simulink model "lht_1280_720"  (R2020a)
settings: Solver=FixedStepDiscrete  StartTime=0.0  StopTime=inf  RelTol=1e-3
InitFcn:
  | setup_parallel_hough_transform;
StopFcn:
  | stop_parallel_hough_accumulator;
values from neighbouring files (symbols this model uses):
  bitsRho = ceil(log2(maxRho*2))    [setup_parallel_hough_transform.m]
  height = 720    [setup_parallel_hough_transform.m]
  inarray = uint8(fi(edge, 0, 1, 0))    [setup_parallel_hough_transform.m]
  width = 1280    [setup_parallel_hough_transform.m]
undefined symbols (not defined in the file or in its folder): fclk, nTheta
libraries: hdlsllib x15, simulink x12, dspsrcs4 x1
(part 1 of 2)
settings Model: DataTypeOverride=Off  SimulationMode=rapid-accelerator  Creator=david  LastModifiedBy=david
settings OptimizationCC: BlockReduction=off  ConditionallyExecuteInputs=off  DefaultParameterBehavior=Inlined
settings DebuggingCC: AlgebraicLoopMsg=error  SingleTaskRateTransMsg=error
settings HardwareCC: ProdBitPerPointer=32  ProdBitPerSizeT=32  ProdBitPerPtrDiffT=32  ProdLargestAtomicFloat=None  ProdIntDivRoundTo=Undefined  ProdEndianess=Unspecified  ProdWordSize=32  ProdHWDeviceType=ASIC/FPGA->ASIC/FPGA  TargetBitPerPointer=64  TargetBitPerSizeT=64  TargetBitPerPtrDiffT=64  TargetLongLongMode=on  TargetIntDivRoundTo=Zero  TargetEndianess=LittleEndian  TargetWordSize=64  TargetHWDeviceType=Custom Processor->MATLAB Host Computer  ProdEqTarget=off

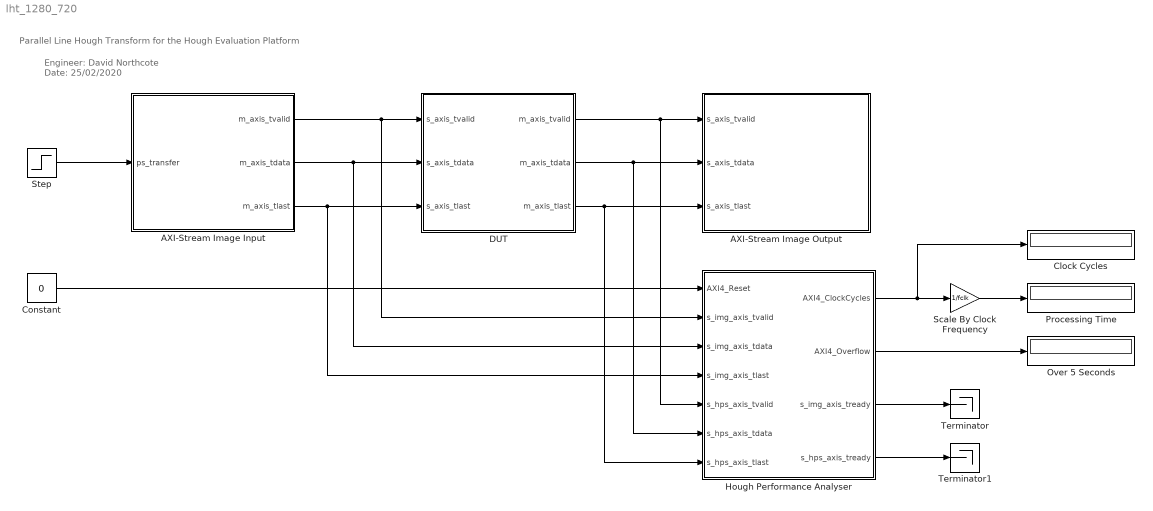
== system lht_1280_720 ==
  note: Engineer: David Northcote
      | Date: 25/02/2020
  note: Parallel Line Hough Transform for the Hough Evaluation Platform
  AXI-Stream Image Input : Subsystem  mask{image=inarray, clk=1/fclk}
      mask prompts: image "Input Image:"; clk "Clock Rate:"
      mask init:
      | [height, width] = size(image);
      mask DialogControl DescGroupVar Prompt: AXI-Stream Image Input
      mask DialogControl DescTextVar Prompt: This block simulates an AXI-Stream image input for interfacing to a hardware accelerator or IP Core.
      mask DialogControl ParameterGroupVar Prompt: Main
  AXI-Stream Image Output : Subsystem  mask{height=ceil(sqrt((height/2)^2+(width/2)^2))*2, width=numel([0:1:179]), clk=1/fclk, d=0}
      mask prompts: height "Image Height:"; width "Image Width:"; clk "Clock Rate:"; d "Frame Capture Number"
      mask DialogControl DescGroupVar Prompt: AXI-Stream Image Output
      mask DialogControl DescTextVar Prompt: Image output using the AXI-Stream interface. Simulates an AXI DMA write channel.
      mask DialogControl ParameterGroupVar Prompt: Main
  Clock Cycles : Display
  Constant : Constant  Value=0  OutDataTypeStr=boolean  SampleTime=1/fclk
  DUT : Subsystem  TreatAsAtomicUnit=on
  Hough Performance Analyser : Subsystem  TreatAsAtomicUnit=on
  Over 5 Seconds : Display
  Processing Time : Display
  Scale By Clock Frequency : Gain  Gain=1/fclk  ParamDataTypeStr=double  OutDataTypeStr=double
  Step : Step  Time=2/150e6  SampleTime=1/fclk
  Terminator : Terminator
  Terminator1 : Terminator
  wires:
  Hough Performance Analyser/1(AXI4_ClockCycles) -> Clock Cycles/1, Scale By Clock Frequency/1
  Scale By Clock Frequency/1 -> Processing Time/1
  DUT/3(m_axis_tlast) -> Hough Performance Analyser/7(s_hps_axis_tlast), AXI-Stream Image Output/3(s_axis_tlast)
  DUT/2(m_axis_tdata) -> Hough Performance Analyser/6(s_hps_axis_tdata), AXI-Stream Image Output/2(s_axis_tdata)
  DUT/1(m_axis_tvalid) -> Hough Performance Analyser/5(s_hps_axis_tvalid), AXI-Stream Image Output/1(s_axis_tvalid)
  AXI-Stream Image Input/3(m_axis_tlast) -> DUT/3(s_axis_tlast), Hough Performance Analyser/4(s_img_axis_tlast)
  AXI-Stream Image Input/1(m_axis_tvalid) -> DUT/1(s_axis_tvalid), Hough Performance Analyser/2(s_img_axis_tvalid)
  AXI-Stream Image Input/2(m_axis_tdata) -> DUT/2(s_axis_tdata), Hough Performance Analyser/3(s_img_axis_tdata)
  Hough Performance Analyser/2(AXI4_Overflow) -> Over 5 Seconds/1
  Constant/1 -> Hough Performance Analyser/1(AXI4_Reset)
  Step/1 -> AXI-Stream Image Input/1(ps_transfer)
  Hough Performance Analyser/4(s_hps_axis_tready) -> Terminator1/1
  Hough Performance Analyser/3(s_img_axis_tready) -> Terminator/1

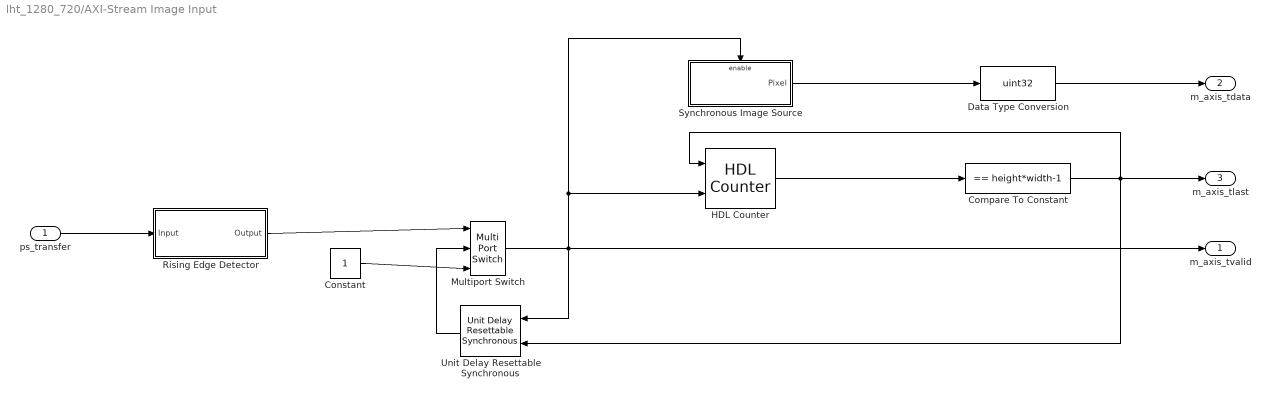
== system lht_1280_720/AXI-Stream Image Input ==
  ps_transfer : Inport
  Compare To Constant : simulink/Logic and Bit Operations/Compare To Constant  relop===  const=height*width-1  OutDataTypeStr=boolean
  Constant : Constant  OutDataTypeStr=boolean  SampleTime=-1
  Data Type Conversion : DataTypeConversion  OutDataTypeStr=uint32
  HDL Counter : hdlsllib/Sources/HDL Counter  CountType=Free running  CountInit=0  CountStep=1  CountMax=width*height-1  CountFromType=Initial value  CountFrom=0  CountResetPort=on  CountLoadPort=off  CountEnbPort=on  CountDirPort=off  CountDataType=Unsigned  CountWordLen=32  CountFracLen=0  CountSampTime=1
  Multiport Switch : MultiPortSwitch  DataPortOrder=Zero-based contiguous  Inputs=2  zeroidx=on
  Rising Edge Detector : Subsystem
  Synchronous Image Source : Subsystem
  Unit Delay Resettable Synchronous : hdlsllib/Discrete/Unit Delay Resettable Synchronous  InitialCondition=0.0  SampleTime=-1
      settings: SourceProductBaseCode=SL
  m_axis_tvalid : Outport
  m_axis_tdata : Outport  Port=2
  m_axis_tlast : Outport  Port=3
  wires:
  Constant/1 -> Multiport Switch/3
  Rising Edge Detector/1(Output) -> Multiport Switch/1
  Unit Delay Resettable Synchronous/1 -> Multiport Switch/2
  ps_transfer/1 -> Rising Edge Detector/1(Input)
  Data Type Conversion/1 -> m_axis_tdata/1
  Compare To Constant/1 -> m_axis_tlast/1, HDL Counter/1, Unit Delay Resettable Synchronous/2
  Multiport Switch/1 -> m_axis_tvalid/1, Synchronous Image Source/Enable, HDL Counter/2, Unit Delay Resettable Synchronous/1
  Synchronous Image Source/1(Pixel) -> Data Type Conversion/1
  HDL Counter/1 -> Compare To Constant/1

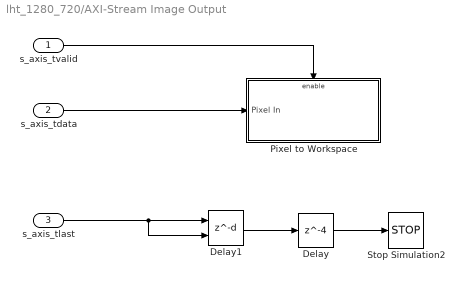
== system lht_1280_720/AXI-Stream Image Output ==
  s_axis_tvalid : Inport
  s_axis_tdata : Inport  Port=2
  s_axis_tlast : Inport  Port=3
  Delay : Delay  DelayLength=4
  Delay1 : Delay  DelayLength=d  ShowEnablePort=on
      settings: InputPortMap=u0,e6
  Pixel to Workspace : Subsystem
  Stop Simulation2 : Stop
  wires:
  Delay/1 -> Stop Simulation2/1
  Delay1/1 -> Delay/1
  s_axis_tlast/1 -> Delay1/1, Delay1/2
  s_axis_tdata/1 -> Pixel to Workspace/1(Pixel In)
  s_axis_tvalid/1 -> Pixel to Workspace/Enable

== system lht_1280_720/DUT ==
  s_axis_tvalid : Inport
  s_axis_tdata : Inport  Port=2
  s_axis_tlast : Inport  Port=3
  LHT : Subsystem
  m_axis_tvalid : Outport  VectorParamsAs1DForOutWhenUnconnected=off
  m_axis_tdata : Outport  Port=2  VectorParamsAs1DForOutWhenUnconnected=off
  m_axis_tlast : Outport  Port=3  VectorParamsAs1DForOutWhenUnconnected=off
  wires:
  s_axis_tdata/1 -> LHT/1(s_tdata)
  s_axis_tvalid/1 -> LHT/2(s_tvalid)
  s_axis_tlast/1 -> LHT/3(s_tlast)
  LHT/3(m_axis_tlast) -> m_axis_tlast/1
  LHT/1(m_axis_tdata) -> m_axis_tdata/1
  LHT/2(m_axis_tvalid) -> m_axis_tvalid/1

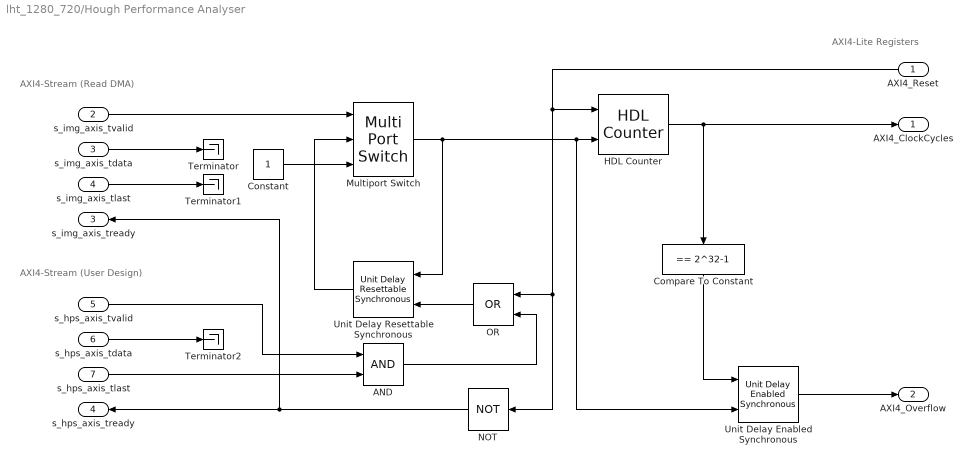
== system lht_1280_720/Hough Performance Analyser ==
  note: AXI4-Stream (Read DMA)
  note: AXI4-Stream (User Design)
  note: AXI4-Lite Registers
  AXI4_Reset : Inport
  s_img_axis_tvalid : Inport  Port=2
  s_img_axis_tdata : Inport  Port=3
  s_img_axis_tlast : Inport  Port=4
  s_hps_axis_tvalid : Inport  Port=5
  s_hps_axis_tdata : Inport  Port=6
  s_hps_axis_tlast : Inport  Port=7
  AND : Logic  IconShape=distinctive  AllPortsSameDT=off  OutDataTypeStr=boolean
  Compare To Constant : simulink/Logic and Bit Operations/Compare To Constant  relop===  const=2^32-1  OutDataTypeStr=boolean
  Constant : Constant  OutDataTypeStr=boolean  SampleTime=-1
  HDL Counter : hdlsllib/Sources/HDL Counter  CountType=Count limited  CountInit=0  CountStep=1  CountMax=2^32-1  CountFromType=Initial value  CountFrom=0  CountResetPort=on  CountLoadPort=off  CountEnbPort=on  CountDirPort=off  CountDataType=Unsigned  CountWordLen=32  CountFracLen=0  CountSampTime=1
  Multiport Switch : MultiPortSwitch  DataPortOrder=Zero-based contiguous  Inputs=2  zeroidx=on
  NOT : Logic  Operator=NOT  IconShape=distinctive  AllPortsSameDT=off  OutDataTypeStr=boolean
  OR : Logic  Operator=OR  IconShape=distinctive  AllPortsSameDT=off  OutDataTypeStr=boolean
  Terminator : Terminator
  Terminator1 : Terminator
  Terminator2 : Terminator
  Unit Delay Enabled Synchronous : hdlsllib/Discrete/Unit Delay Enabled Synchronous  InitialCondition=0.0  SampleTime=-1
      settings: SourceProductBaseCode=SL
  Unit Delay Resettable Synchronous : hdlsllib/Discrete/Unit Delay Resettable Synchronous  InitialCondition=0.0  SampleTime=-1
      settings: SourceProductBaseCode=SL
  AXI4_ClockCycles : Outport
  AXI4_Overflow : Outport  Port=2
  s_img_axis_tready : Outport  Port=3
  s_hps_axis_tready : Outport  Port=4
  wires:
  NOT/1 -> s_hps_axis_tready/1, s_img_axis_tready/1
  s_hps_axis_tvalid/1 -> AND/1
  s_hps_axis_tlast/1 -> AND/2
  AND/1 -> OR/2
  s_img_axis_tvalid/1 -> Multiport Switch/1
  OR/1 -> Unit Delay Resettable Synchronous/2
  s_img_axis_tlast/1 -> Terminator1/1
  AXI4_Reset/1 -> HDL Counter/1, OR/1, NOT/1
  s_img_axis_tdata/1 -> Terminator/1
  s_hps_axis_tdata/1 -> Terminator2/1
  HDL Counter/1 -> AXI4_ClockCycles/1, Compare To Constant/1
  Unit Delay Enabled Synchronous/1 -> AXI4_Overflow/1
  Compare To Constant/1 -> Unit Delay Enabled Synchronous/1
  Multiport Switch/1 -> HDL Counter/2, Unit Delay Enabled Synchronous/2, Unit Delay Resettable Synchronous/1
  Unit Delay Resettable Synchronous/1 -> Multiport Switch/2
  Constant/1 -> Multiport Switch/3

== system lht_1280_720/AXI-Stream Image Input/Rising Edge Detector ==
  Input : Inport
  AND : Logic  IconShape=distinctive  AllPortsSameDT=off  OutDataTypeStr=boolean
  Delay : Delay  DelayLength=1
  NOT : Logic  Operator=NOT  IconShape=distinctive  AllPortsSameDT=off  OutDataTypeStr=boolean
  Output : Outport  VectorParamsAs1DForOutWhenUnconnected=off
  wires:
  AND/1 -> Output/1
  Delay/1 -> AND/1
  Input/1 -> NOT/1, AND/2
  NOT/1 -> Delay/1

== system lht_1280_720/AXI-Stream Image Input/Synchronous Image Source ==
  Enable : EnablePort
  Signal From Workspace : dspsrcs4/Signal From Workspace  X=reshape(image', [height*width, 1])  Ts=clk  nsamps=1  OutputAfterFinalValue=Cyclic repetition  ignoreOrWarnInputAndFrameLengths=off  OutputFrames=off
  Pixel : Outport
  wires:
  Signal From Workspace/1 -> Pixel/1

== system lht_1280_720/AXI-Stream Image Output/Pixel to Workspace ==
  Pixel In : Inport
  Enable : EnablePort
  To Workspace : ToWorkspace  VariableName=simout  SampleTime=-1
      settings: MaxDataPoints=height*width  Save2DSignal=2-D array (concatenate along first dimension)
  wires:
  Pixel In/1 -> To Workspace/1

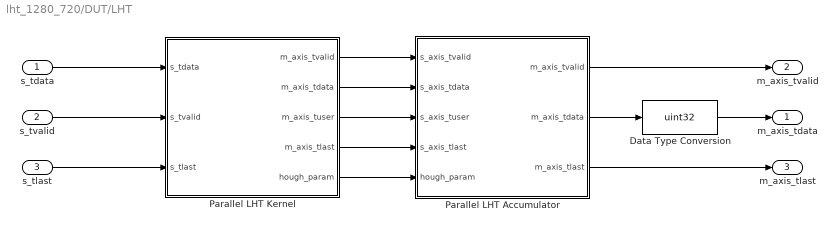
== system lht_1280_720/DUT/LHT ==
  s_tdata : Inport
  s_tvalid : Inport  Port=2
  s_tlast : Inport  Port=3
  Data Type Conversion : DataTypeConversion  OutDataTypeStr=uint32
  Parallel LHT Accumulator : Subsystem  mask{height=height, width=width, theta=[0:1:179]}
      mask prompts: height "Image Height:"; width "Image Width:"; theta "Orientations:"
      mask init:
      | maxRho = ceil(sqrt((height/2)^2+(width/2)^2));
      | nRho = maxRho*2;
      | [~, nTheta] = size(theta);
      mask DialogControl ParameterGroupVar Prompt: Main
  Parallel LHT Kernel : Subsystem
  m_axis_tdata : Outport  VectorParamsAs1DForOutWhenUnconnected=off
  m_axis_tvalid : Outport  Port=2  VectorParamsAs1DForOutWhenUnconnected=off
  m_axis_tlast : Outport  Port=3  VectorParamsAs1DForOutWhenUnconnected=off
  wires:
  s_tdata/1 -> Parallel LHT Kernel/1(s_tdata)
  s_tvalid/1 -> Parallel LHT Kernel/2(s_tvalid)
  s_tlast/1 -> Parallel LHT Kernel/3(s_tlast)
  Parallel LHT Kernel/1(m_axis_tvalid) -> Parallel LHT Accumulator/1(s_axis_tvalid)
  Parallel LHT Kernel/2(m_axis_tdata) -> Parallel LHT Accumulator/2(s_axis_tdata)
  Parallel LHT Kernel/4(m_axis_tlast) -> Parallel LHT Accumulator/4(s_axis_tlast)
  Parallel LHT Kernel/3(m_axis_tuser) -> Parallel LHT Accumulator/3(s_axis_tuser)
  Parallel LHT Kernel/5(hough_param) -> Parallel LHT Accumulator/5(hough_param)
  Parallel LHT Accumulator/2(m_axis_tdata) -> Data Type Conversion/1
  Parallel LHT Accumulator/1(m_axis_tvalid) -> m_axis_tvalid/1
  Parallel LHT Accumulator/3(m_axis_tlast) -> m_axis_tlast/1
  Data Type Conversion/1 -> m_axis_tdata/1

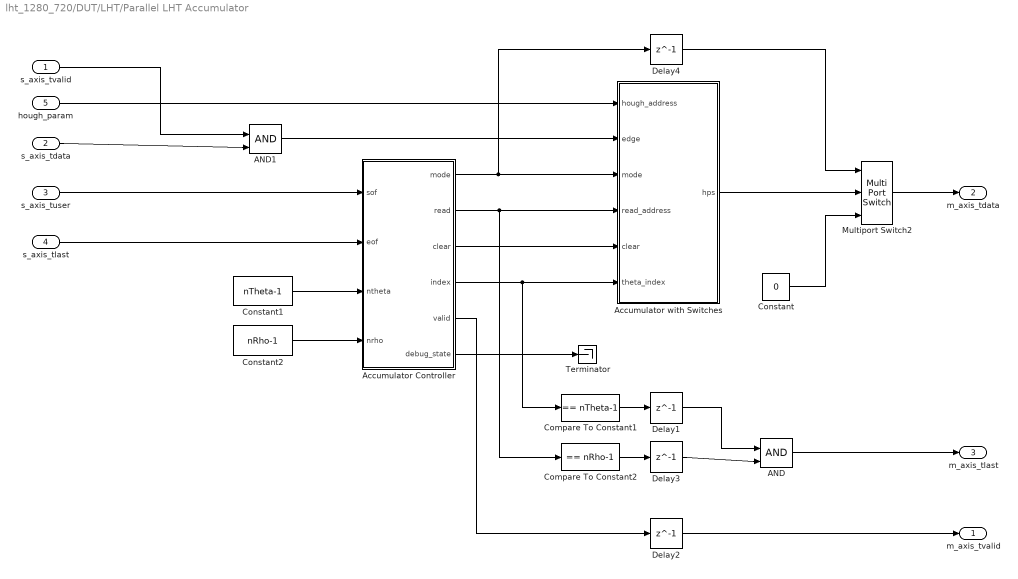
== system lht_1280_720/DUT/LHT/Parallel LHT Accumulator ==
  s_axis_tvalid : Inport
  s_axis_tdata : Inport  Port=2
  s_axis_tuser : Inport  Port=3
  s_axis_tlast : Inport  Port=4
  hough_param : Inport  Port=5
  AND : Logic  IconShape=distinctive  AllPortsSameDT=off  OutDataTypeStr=boolean
  AND1 : Logic  IconShape=distinctive  AllPortsSameDT=off  OutDataTypeStr=boolean
  Accumulator Controller : MATLAB Function  TreatAsAtomicUnit=on
  Accumulator with Switches : Subsystem
  Compare To Constant1 : simulink/Logic and Bit Operations/Compare To Constant  relop===  const=nTheta-1  OutDataTypeStr=boolean
  Compare To Constant2 : simulink/Logic and Bit Operations/Compare To Constant  relop===  const=nRho-1  OutDataTypeStr=boolean
  Constant : Constant  Value=0  OutDataTypeStr=fixdt(0, ceil(log2(2*maxRho)), 0)  SampleTime=-1
  Constant1 : Constant  Value=nTheta-1  OutDataTypeStr=uint16  SampleTime=-1
  Constant2 : Constant  Value=nRho-1  OutDataTypeStr=uint16  SampleTime=-1
  Delay{1..4} (4 alike) : Delay  DelayLength=1
  Multiport Switch2 : MultiPortSwitch  DataPortOrder=Zero-based contiguous  Inputs=2  zeroidx=on
  Terminator : Terminator
  m_axis_tvalid : Outport
  m_axis_tdata : Outport  Port=2
  m_axis_tlast : Outport  Port=3
  wires:
  s_axis_tlast/1 -> Accumulator Controller/2(eof)
  Accumulator Controller/6(debug_state) -> Terminator/1
  Delay4/1 -> Multiport Switch2/1
  Delay2/1 -> m_axis_tvalid/1
  Accumulator Controller/5(valid) -> Delay2/1
  Constant/1 -> Multiport Switch2/3
  Accumulator with Switches/1(hps) -> Multiport Switch2/2
  Multiport Switch2/1 -> m_axis_tdata/1
  s_axis_tvalid/1 -> AND1/1
  AND1/1 -> Accumulator with Switches/2(edge)
  s_axis_tdata/1 -> AND1/2
  hough_param/1 -> Accumulator with Switches/1(hough_address)
  s_axis_tuser/1 -> Accumulator Controller/1(sof)
  Constant2/1 -> Accumulator Controller/4(nrho)
  Compare To Constant2/1 -> Delay3/1
  Accumulator Controller/4(index) -> Compare To Constant1/1, Accumulator with Switches/6(theta_index)
  Constant1/1 -> Accumulator Controller/3(ntheta)
  Accumulator Controller/2(read) -> Accumulator with Switches/4(read_address), Compare To Constant2/1
  Accumulator Controller/1(mode) -> Accumulator with Switches/3(mode), Delay4/1
  Accumulator Controller/3(clear) -> Accumulator with Switches/5(clear)
  Compare To Constant1/1 -> Delay1/1
  Delay3/1 -> AND/2
  Delay1/1 -> AND/1
  AND/1 -> m_axis_tlast/1

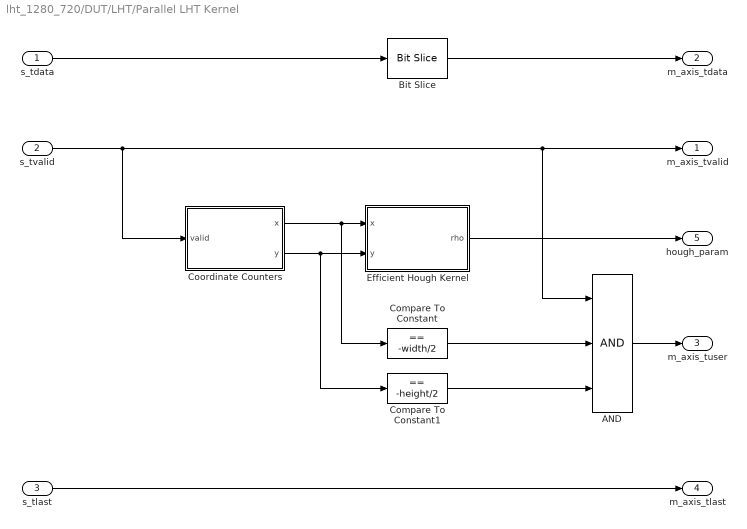
== system lht_1280_720/DUT/LHT/Parallel LHT Kernel ==
  s_tdata : Inport
  s_tvalid : Inport  Port=2
  s_tlast : Inport  Port=3
  AND : Logic  Inputs=3  IconShape=distinctive  AllPortsSameDT=off  OutDataTypeStr=boolean
  Bit Slice : hdlsllib/Logic and Bit Operations/Bit Slice  lidx=0  ridx=0
      settings: SourceProductBaseCode=SL
  Compare To Constant : simulink/Logic and Bit Operations/Compare To Constant  relop===  const=-width/2  OutDataTypeStr=boolean
  Compare To Constant1 : simulink/Logic and Bit Operations/Compare To Constant  relop===  const=-height/2  OutDataTypeStr=boolean
  Coordinate Counters : Subsystem
  Efficient Hough Kernel : Subsystem  mask{height=height, width=width}
      mask prompts: height "Image Height:"; width "Image Width:"
      mask init:
      | theta = [0:1:179];
      | 
      | maxRho = ceil(sqrt((height/2)^2+(width/2)^2));
      | [~, nTheta] = size(theta);
      | nRho = maxRho*2;
      mask DialogControl DescGroupVar Prompt: Efficient Hough Kernel
      mask DialogControl DescTextVar Prompt: The efficient Hough kernel uses look ahead and symmetric techniques to optimise DSP consumption.
  m_axis_tvalid : Outport  VectorParamsAs1DForOutWhenUnconnected=off
  m_axis_tdata : Outport  Port=2  VectorParamsAs1DForOutWhenUnconnected=off
  m_axis_tuser : Outport  Port=3  VectorParamsAs1DForOutWhenUnconnected=off
  m_axis_tlast : Outport  Port=4  VectorParamsAs1DForOutWhenUnconnected=off
  hough_param : Outport  Port=5  VectorParamsAs1DForOutWhenUnconnected=off
  wires:
  s_tlast/1 -> m_axis_tlast/1
  Compare To Constant/1 -> AND/2
  AND/1 -> m_axis_tuser/1
  Coordinate Counters/1(x) -> Compare To Constant/1, Efficient Hough Kernel/1(x)
  s_tvalid/1 -> m_axis_tvalid/1, AND/1, Coordinate Counters/1(valid)
  Coordinate Counters/2(y) -> Compare To Constant1/1, Efficient Hough Kernel/2(y)
  Compare To Constant1/1 -> AND/3
  Efficient Hough Kernel/1(rho) -> hough_param/1
  s_tdata/1 -> Bit Slice/1
  Bit Slice/1 -> m_axis_tdata/1

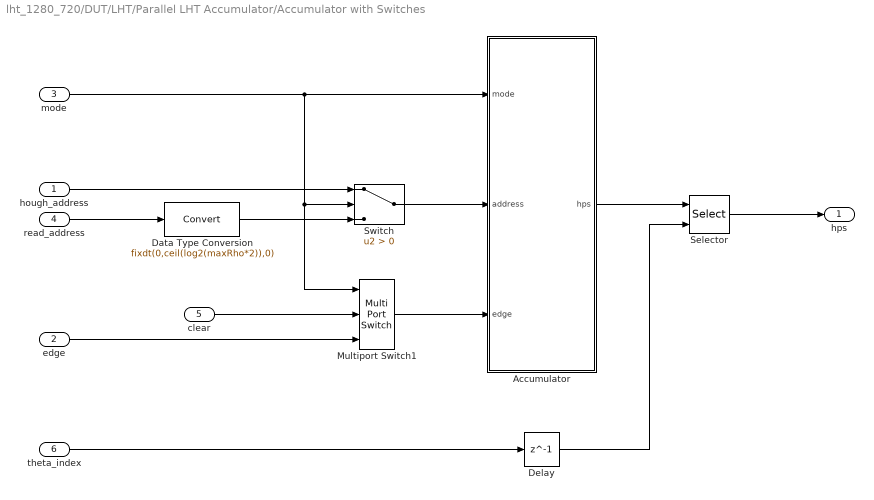
== system lht_1280_720/DUT/LHT/Parallel LHT Accumulator/Accumulator with Switches ==
  hough_address : Inport
  edge : Inport  Port=2
  mode : Inport  Port=3
  read_address : Inport  Port=4
  clear : Inport  Port=5
  theta_index : Inport  Port=6
  Accumulator : Subsystem
  Data Type Conversion : DataTypeConversion  OutDataTypeStr=fixdt(0,ceil(log2(maxRho*2)),0)
  Delay : Delay  DelayLength=1
  Multiport Switch1 : MultiPortSwitch  DataPortOrder=Zero-based contiguous  Inputs=2  zeroidx=on
  Selector : Selector  NumberOfDimensions=2  IndexMode=Zero-based  InputPortWidth=3  IndexOptions=Index vector (dialog),Index vector (port)  Indices=0,0  OutputSizes=1,1
  Switch : Switch  Criteria=u2 > Threshold
  hps : Outport
  wires:
  Delay/1 -> Selector/2
  Data Type Conversion/1 -> Switch/3
  clear/1 -> Multiport Switch1/2
  edge/1 -> Multiport Switch1/3
  Selector/1 -> hps/1
  theta_index/1 -> Delay/1
  hough_address/1 -> Switch/1
  Multiport Switch1/1 -> Accumulator/3(edge)
  Switch/1 -> Accumulator/2(address)
  read_address/1 -> Data Type Conversion/1
  mode/1 -> Accumulator/1(mode), Multiport Switch1/1, Switch/2
  Accumulator/1(hps) -> Selector/1

== system lht_1280_720/DUT/LHT/Parallel LHT Kernel/Coordinate Counters ==
  valid : Inport
  AND : Logic  IconShape=distinctive  AllPortsSameDT=off  OutDataTypeStr=boolean
  Compare To Constant : simulink/Logic and Bit Operations/Compare To Constant  relop===  const=width/2-1  OutDataTypeStr=boolean
  X Counter : hdlsllib/Sources/HDL Counter  CountType=Count limited  CountInit=-width/2  CountStep=1  CountMax=width/2-1  CountFromType=Initial value  CountFrom=-width/2  CountResetPort=off  CountLoadPort=off  CountEnbPort=on  CountDirPort=off  CountDataType=Signed  CountWordLen=ceil(log2(width/2)) + 1  CountFracLen=0  CountSampTime=1
  Y Counter : hdlsllib/Sources/HDL Counter  CountType=Count limited  CountInit=-height/2  CountStep=1  CountMax=height/2-1  CountFromType=Initial value  CountFrom=-height/2  CountResetPort=off  CountLoadPort=off  CountEnbPort=on  CountDirPort=off  CountDataType=Signed  CountWordLen=ceil(log2(height/2)) + 1  CountFracLen=0  CountSampTime=1
  x : Outport  VectorParamsAs1DForOutWhenUnconnected=off
  y : Outport  Port=2  VectorParamsAs1DForOutWhenUnconnected=off
  wires:
  valid/1 -> AND/2, X Counter/1
  X Counter/1 -> x/1, Compare To Constant/1
  Y Counter/1 -> y/1
  AND/1 -> Y Counter/1
  Compare To Constant/1 -> AND/1

== system lht_1280_720/DUT/LHT/Parallel LHT Kernel/Efficient Hough Kernel ==
  x : Inport
  y : Inport  Port=2
  Add : Sum  OutDataTypeStr=fixdt(0, ceil(log2(2*maxRho+1)), 0)  RndMeth=Round
  Constant : Constant  Value=maxRho  OutDataTypeStr=fixdt(0, ceil(log2(maxRho + 1)), 0)  SampleTime=-1
  Look Ahead Hough : Subsystem
  Symmetric Kernel : Subsystem
  rho : Outport  VectorParamsAs1DForOutWhenUnconnected=off
  wires:
  Look Ahead Hough/1(ysin) -> Symmetric Kernel/2(ysin)
  y/1 -> Look Ahead Hough/2(y)
  Symmetric Kernel/1(rho) -> Add/2
  Add/1 -> rho/1
  Constant/1 -> Add/1
  x/1 -> Symmetric Kernel/1(x), Look Ahead Hough/1(x)

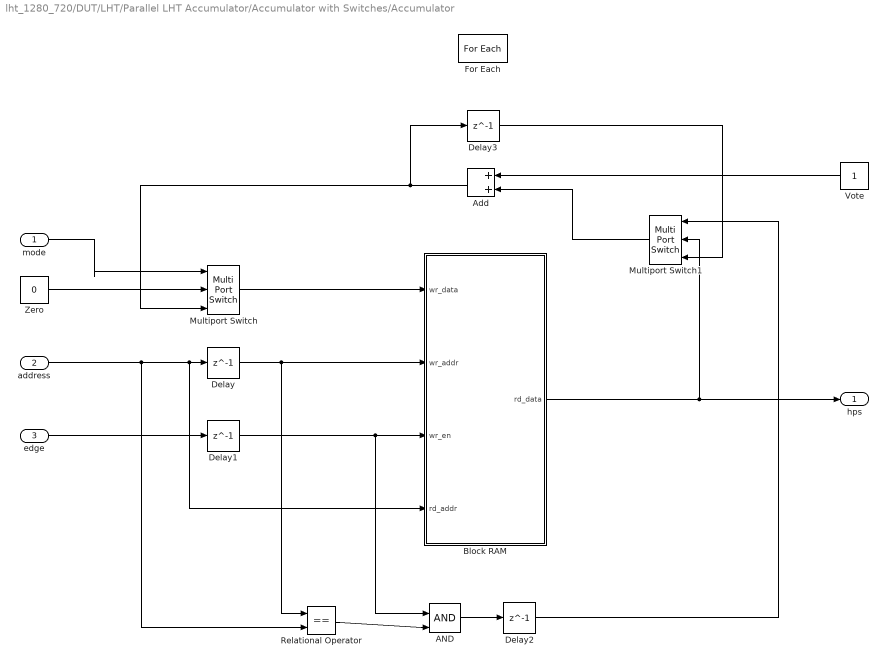
== system lht_1280_720/DUT/LHT/Parallel LHT Accumulator/Accumulator with Switches/Accumulator ==
  mode : Inport
  address : Inport  Port=2  Partition=on  PartitionDimension=2  PartitionWidth=1  PartitionOffset=0
  edge : Inport  Port=3
  AND : Logic  IconShape=distinctive  AllPortsSameDT=off  OutDataTypeStr=boolean
  Add : Sum  OutDataTypeStr=fixdt(0, ceil(log2(maxRho*2)), 0)
  Block RAM : Subsystem  Variant=on  VariantControlMode=Label  VariantControl=Variant1  LabelModeActiveChoice=other_bits
  Delay{,1..3} (4 alike) : Delay  DelayLength=1
  For Each : ForEach  DisableCoverage=on
  Multiport Switch : MultiPortSwitch  DataPortOrder=Zero-based contiguous  Inputs=2  zeroidx=on
  Multiport Switch1 : MultiPortSwitch  DataPortOrder=Zero-based contiguous  Inputs=2  zeroidx=on
  Relational Operator : RelationalOperator  Operator===  OutDataTypeStr=boolean  RndMeth=Simplest
  Vote : Constant  OutDataTypeStr=fixdt(0,1,0)  SampleTime=-1
  Zero : Constant  Value=0  OutDataTypeStr=fixdt(0,1,0)  SampleTime=-1
  hps : Outport  ConcatenationDimension=2
  wires:
  Block RAM/1(rd_data) -> hps/1, Multiport Switch1/2
  Multiport Switch/1 -> Block RAM/1(wr_data)
  mode/1 -> Multiport Switch/1
  edge/1 -> Delay1/1
  Zero/1 -> Multiport Switch/2
  Delay3/1 -> Multiport Switch1/3
  Vote/1 -> Add/1
  Multiport Switch1/1 -> Add/2
  Add/1 -> Delay3/1, Multiport Switch/3
  Delay1/1 -> Block RAM/3(wr_en), AND/1
  AND/1 -> Delay2/1
  address/1 -> Relational Operator/2, Delay/1, Block RAM/4(rd_addr)
  Delay2/1 -> Multiport Switch1/1
  Delay/1 -> Block RAM/2(wr_addr), Relational Operator/1
  Relational Operator/1 -> AND/2

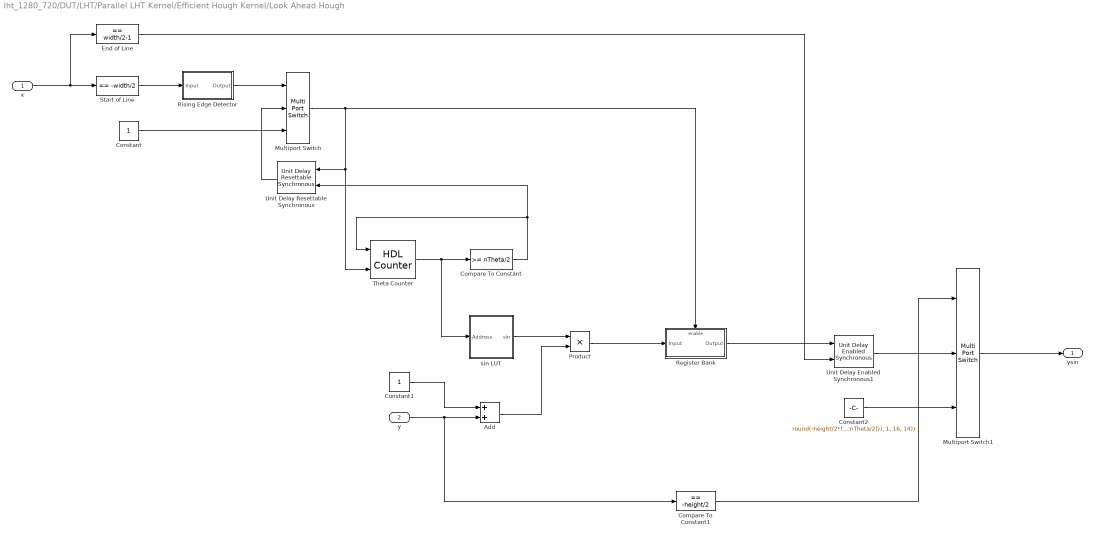
== system lht_1280_720/DUT/LHT/Parallel LHT Kernel/Efficient Hough Kernel/Look Ahead Hough ==
  x : Inport
  y : Inport  Port=2
  Add : Sum  OutDataTypeStr=fixdt(1,ceil(log2(height)),0)
  Compare To Constant : simulink/Logic and Bit Operations/Compare To Constant  relop=>=  const=nTheta/2  OutDataTypeStr=boolean
  Compare To Constant1 : simulink/Logic and Bit Operations/Compare To Constant  relop===  const=-height/2  OutDataTypeStr=boolean
  Constant : Constant  OutDataTypeStr=boolean  SampleTime=-1
  Constant1 : Constant  OutDataTypeStr=fixdt(1, ceil(log2(height)), 0);  SampleTime=-1
  Constant2 : Constant  Value=round(-height/2*fi(sin(deg2rad([0:1:nTheta/2])), 1, 16, 14))  OutDataTypeStr=fixdt(1,ceil(log2(height)),0)  SampleTime=-1
  End of Line : simulink/Logic and Bit Operations/Compare To Constant  relop===  const=width/2-1  OutDataTypeStr=boolean
  Multiport Switch : MultiPortSwitch  DataPortOrder=Zero-based contiguous  Inputs=2  zeroidx=on
  Multiport Switch1 : MultiPortSwitch  DataPortOrder=Zero-based contiguous  Inputs=2  zeroidx=on
  Product : Product  OutDataTypeStr=fixdt(1, ceil(log2(height)), 0);  RndMeth=Round
  Register Bank : Subsystem
  Rising Edge Detector : Subsystem
  Start of Line : simulink/Logic and Bit Operations/Compare To Constant  relop===  const=-width/2  OutDataTypeStr=boolean
  Theta Counter : hdlsllib/Sources/HDL Counter  CountType=Count limited  CountInit=0  CountStep=1  CountMax=nTheta/2  CountFromType=Initial value  CountFrom=0  CountResetPort=on  CountLoadPort=off  CountEnbPort=on  CountDirPort=off  CountDataType=Unsigned  CountWordLen=ceil(log2(nTheta))  CountFracLen=0  CountSampTime=1
  Unit Delay Enabled Synchronous1 : hdlsllib/Discrete/Unit Delay Enabled Synchronous  InitialCondition=0.0  SampleTime=-1
      settings: SourceProductBaseCode=SL
  Unit Delay Resettable Synchronous : hdlsllib/Discrete/Unit Delay Resettable Synchronous  InitialCondition=0.0  SampleTime=-1
      settings: SourceProductBaseCode=SL
  sin LUT : Subsystem
  ysin : Outport  VectorParamsAs1DForOutWhenUnconnected=off
  wires:
  x/1 -> End of Line/1, Start of Line/1
  Start of Line/1 -> Rising Edge Detector/1(Input)
  Multiport Switch/1 -> Register Bank/Enable, Unit Delay Resettable Synchronous/1, Theta Counter/2
  Unit Delay Resettable Synchronous/1 -> Multiport Switch/2
  Constant/1 -> Multiport Switch/3
  Theta Counter/1 -> sin LUT/1(Address), Compare To Constant/1
  Constant1/1 -> Add/1
  Rising Edge Detector/1(Output) -> Multiport Switch/1
  Add/1 -> Product/2
  Multiport Switch1/1 -> ysin/1
  Constant2/1 -> Multiport Switch1/3
  Compare To Constant1/1 -> Multiport Switch1/1
  Product/1 -> Register Bank/1(Input)
  y/1 -> Add/2, Compare To Constant1/1
  Compare To Constant/1 -> Unit Delay Resettable Synchronous/2, Theta Counter/1
  Unit Delay Enabled Synchronous1/1 -> Multiport Switch1/2
  End of Line/1 -> Unit Delay Enabled Synchronous1/2
  Register Bank/1(Output) -> Unit Delay Enabled Synchronous1/1
  sin LUT/1(sin) -> Product/1

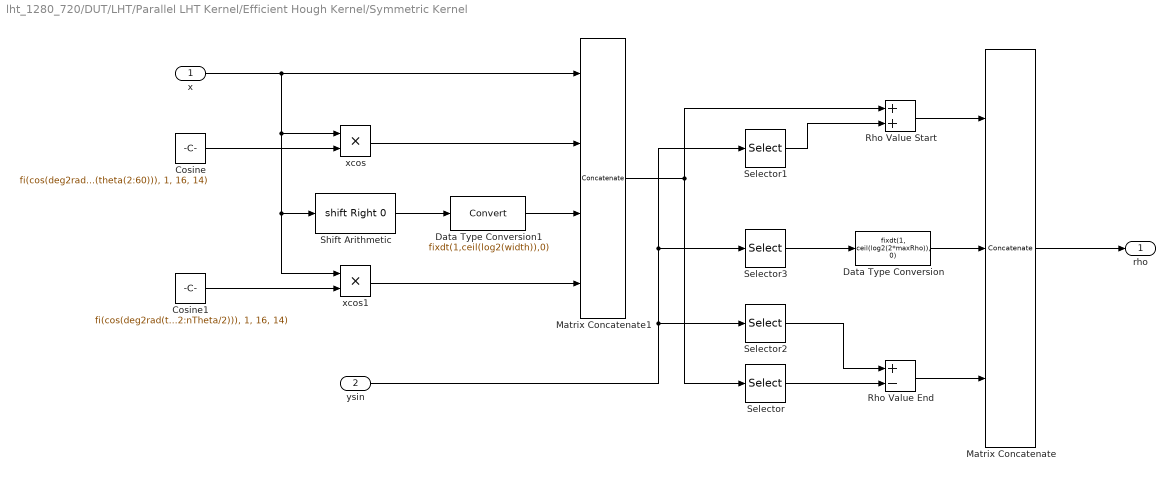
== system lht_1280_720/DUT/LHT/Parallel LHT Kernel/Efficient Hough Kernel/Symmetric Kernel ==
  x : Inport
  ysin : Inport  Port=2
  Cosine : Constant  Value=fi(cos(deg2rad(theta(2:60))), 1, 16, 14)  VectorParams1D=off  OutDataTypeStr=fixdt(1,16,14)  SampleTime=-1
  Cosine1 : Constant  Value=fi(cos(deg2rad(theta(62:nTheta/2))), 1, 16, 14)  VectorParams1D=off  OutDataTypeStr=fixdt(1,16,14)  SampleTime=-1
  Data Type Conversion : DataTypeConversion  OutDataTypeStr=fixdt(1, ceil(log2(2*maxRho)), 0)  RndMeth=Round
  Data Type Conversion1 : DataTypeConversion  OutDataTypeStr=fixdt(1,ceil(log2(width)),0)  RndMeth=Round
  Matrix Concatenate : Concatenate  NumInputs=3  Mode=Multidimensional array  ConcatenateDimension=2
  Matrix Concatenate1 : Concatenate  NumInputs=4  Mode=Multidimensional array  ConcatenateDimension=2
  Rho Value End : Sum  Inputs=+-  OutDataTypeStr=fixdt(1, ceil(log2(2*maxRho)), 0)  RndMeth=Round
  Rho Value Start : Sum  OutDataTypeStr=fixdt(1, ceil(log2(2*maxRho)), 0)  RndMeth=Round
  Selector : Selector  IndexMode=Zero-based  InputPortWidth=nTheta/2  IndexOptions=Index vector (dialog)  Indices=uint32([nTheta/2-1:-1:1])  OutputSizes=1
  Selector1 : Selector  IndexMode=Zero-based  InputPortWidth=nTheta/2+1  IndexOptions=Index vector (dialog)  Indices=[0:1:nTheta/2-1]  OutputSizes=1
  Selector2 : Selector  IndexMode=Zero-based  InputPortWidth=nTheta/2+1  IndexOptions=Index vector (dialog)  Indices=uint32([nTheta/2-1:-1:1])  OutputSizes=1
  Selector3 : Selector  IndexMode=Zero-based  InputPortWidth=nTheta/2+1  IndexOptions=Index vector (dialog)  Indices=uint32([nTheta/2])  OutputSizes=1
  Shift Arithmetic : ArithShift  BinPtShiftNumber=-1  BitShiftDirection=Right
  xcos : Product  OutDataTypeStr=fixdt(1,ceil(log2(width)),0)  RndMeth=Round
  xcos1 : Product  OutDataTypeStr=fixdt(1,ceil(log2(width)),0)  RndMeth=Round
  rho : Outport  VectorParamsAs1DForOutWhenUnconnected=off
  wires:
  Rho Value End/1 -> Matrix Concatenate/3
  Selector/1 -> Rho Value End/2
  Matrix Concatenate/1 -> rho/1
  Rho Value Start/1 -> Matrix Concatenate/1
  Selector3/1 -> Data Type Conversion/1
  Selector1/1 -> Rho Value Start/2
  Selector2/1 -> Rho Value End/1
  Cosine/1 -> xcos/2
  ysin/1 -> Selector2/1, Selector3/1, Selector1/1
  Data Type Conversion/1 -> Matrix Concatenate/2
  xcos/1 -> Matrix Concatenate1/2
  Matrix Concatenate1/1 -> Rho Value Start/1, Selector/1
  xcos1/1 -> Matrix Concatenate1/4
  Cosine1/1 -> xcos1/2
  x/1 -> xcos1/1, Shift Arithmetic/1, xcos/1, Matrix Concatenate1/1
  Shift Arithmetic/1 -> Data Type Conversion1/1
  Data Type Conversion1/1 -> Matrix Concatenate1/3

== system lht_1280_720/DUT/LHT/Parallel LHT Accumulator/Accumulator with Switches/Accumulator/Block RAM ==
  wr_data : Inport
  wr_addr : Inport  Port=2
  wr_en : Inport  Port=3
  rd_addr : Inport  Port=4
  Simple Dual Port RAM : Subsystem  VariantControl=9_bits
  Simple Dual Port RAM Generator : Subsystem  VariantControl=other_bits  mask{b=bitsRho, d=maxRho*2, b_hidden=36, d_hidden=1470}
      mask prompts: b "Data width:"; d "Depth:"
      mask init:
      | if d == d_hidden
      |     return
      | end
      | 
      | set_param(gcb, 'd_hidden', int2str(d));
      | 
      | % Xilinx RAM Initialisation
      | xl_config = [512, 72;
      |             1024, 36;
      |             2048, 18;
      |             4096, 9;
      |             8192, 4;
      |             16384, 2;
      |             32768, 1];
      | 
      | % Get length of Xilinx Configuration
      | sizeram = size(xl_config);
      |         
      | % Get the RAM Configuration based on the data width
      | for i = 1:sizeram(1)
      |     if b <= xl_config(i, 2)
      |         a = xl_config(i, :);
      |     end
      | end
      | 
      | % Get number of BRAM required (including half BRAM)
      | numbram = ceil((d/a(1))/0.5)*0.5;
      | fullbram = floor(numbram); % Integer
      | halfbram = (numbram-floor(numbram)) ~= 0; % Boolean
      | 
      | % Get all blocks and delete everything excepts ports
      | H = get(find_system(gcb, 'FindAll', 'on', 'type', 'block'));
      | todelete = setdiff(strcat(repmat({[gcb '/']}, numel(H.Blocks), 1),  H.Blocks),...
      |     strcat(repmat({[gcb '/']}, 5, 1),...
      |     {'wr_data'; 'wr_addr'; 'wr_en'; 'rd_addr'; 'rd_data'}));
      | delete_block(todelete);
      | 
      | % Delete lines
      | for i = 1:numel(H.Lines)
      |     delete_line(H.Lines(i).Handle)
      | end
      | 
      | % Generate full BRAMs
      | y = 0;
      | 
      | % If there is only one ram then the write enable should be directly
      | % connected to the first ram write enable. Else, the write address must be sliced
      | % and the upper bound (over a(2)) compared to zero. This will indicate if
      | % the first ram is the one to be written/read from.
      | 
      | % Common to both implementations
      | % Write Address Slice
      | add_block('hdlsllib/Logic and Bit Operations/Bit Slice',...
      |         [gcb, '/wr_address'], 'Position',...
      |         [160 130 250 170]);
      | % Set bitslice parameters
      | set_param([gcb, '/wr_address'],...
      |     'lidx', int2str(log2(a(1))-1));
      | set_param([gcb, '/wr_address'],...
      |     'ridx', int2str(0));
      | 
      | % Read Address Slice
      | add_block('hdlsllib/Logic and Bit Operations/Bit Slice',...
      |         [gcb, '/rd_address'], 'Position',...
      |         [160 330 250 370]);
      | % Set bitslice parameters
      | set_param([gcb, '/rd_address'],...
      |     'lidx', int2str(log2(a(1))-1));
      | set_param([gcb, '/rd_address'],...
      |     'ridx', int2str(0));
      | 
      | if ceil(numbram) == 1
      |     
      |     i = 1;
      |     
      |     % Set bitslice parameters
      |     set_param([gcb, '/rd_address'],...
      |         'lidx', int2str(ceil(log2(d))-1));
      |     set_param([gcb, '/wr_address'],...
      |         'lidx', int2str(ceil(log2(d))-1));
      |     
      |     % Add Simple RAM
      |     add_block('hdlsllib/HDL RAMs/Simple Dual Port RAM',...
      |         [gcb, '/simple_ram_', int2str(i-1)], 'Position',...
      |         [635 0+600*y 635+200 400+600*y]);
      | 
      |     % Set RAM parameters
      |     set_param([gcb, '/simple_ram_', int2str(i-1)],...
      |         'ram_size', int2str(ceil(log2(d))));
      | 
      |     % Connect "wr_data" to "simple_ram_i"
      |     add_line(gcb, ['wr_data/1'], ['simple_ram_', int2str(i-1), '/1'],...
      |         'autorouting', 'on');
      |     
      |     % Connect "wr_addr" to "wr_address"
      |     add_line(gcb, ['wr_addr/1'], ['wr_address/1'],...
      |         'autorouting', 'on');
      | 
      |     % Connect "wr_address" to "simple_ram_i"
      |     add_line(gcb, ['wr_address/1'], ['simple_ram_', int2str(i-1), '/2'],...
      |         'autorouting', 'on');
      | 
      |     % Connect "wr_en" to "simple_ram_i"
      |     add_line(gcb, ['wr_en/1'], ['simple_ram_', int2str(i-1), '/3'],...
      |         'autorouting', 'on');
      |     
      |     % Connect "rd_addr" to "rd_address"
      |     add_line(gcb, ['rd_addr/1'], ['rd_address/1'],...
      |         'autorouting', 'on');
      | 
      |     % Connect "rd_address" to "simple_ram_i"
      |     add_line(gcb, ['rd_address/1'], ['simple_ram_', int2str(i-1), '/4'],...
      |         'autorouting', 'on');
      |     
      |     % Connect "simple_ram_i" to "rd_data"
      |     add_line(gcb, ['simple_ram_', int2str(i-1), '/1'], ['rd_data/1'],...
      |         'autorouting', 'on');
      | 
      | else
      |     
      |     % Multiport Switch
      |     add_block('hdlsllib/Signal Routing/Multiport Switch',...
      |         [gcb, '/multiport_switch'], 'Position',...
      |         [1340 146 1405 250]);
      |     % Set multiport switch parameters
      |     set_param([gcb, '/multiport_switch'],...
      |         'Inputs', int2str(ceil(numbram)));
      |     set_param([gcb, '/multiport_switch'],...
      |         'DataPortOrder', 'Zero-based contiguous');
      | 
      |     % Add Constant Zero
      |     add_block('hdlsllib/Sources/Constant',...
      |         [gcb, '/zero'], 'Position',...
      |         [425 -65 455 -35]);
      |     set_param([gcb, '/zero'],...
      |         'Value', int2str(0));
      |     set_param([gcb, '/zero'],...
      |         'OutDataTypeStr', ['fixdt(0, ', int2str(ceil(numbram)), ', 0)']);
      | 
      |     % Add Vector Concatenate
      |     add_block('hdlsllib/Signal Routing/Vector Concatenate',...
      |         [gcb, '/vector_concatenate'], 'Position',...
      |         [1015, -113, 1025, 38]);
      |     set_param([gcb, '/vector_concatenate'],...
      |         'NumInputs', int2str(ceil(numbram)));
      | 
      |     % Add Bitwise-OR
      |     add_block('hdlsllib/Logic and Bit Operations/Bitwise Operator',...
      |         [gcb, '/bitwise_or'], 'Position',...
      |         [1165, -54, 1205, -16]);
      |     set_param([gcb, '/bitwise_or'],...
      |         'logicop', 'OR');
      |     set_param([gcb, '/bitwise_or'],...
      |         'UseBitMask', 0);
      |     set_param([gcb, '/bitwise_or'],...
      |         'NumInputPorts', int2str(1));
      | 
      |     % Add delay for bram access
      |     add_block('hdlsllib/Discrete/Delay',...
      |         [gcb, '/delay'], 'Position',...
      |         [1248, 60, 1282, 95]);
      |     set_param([gcb, '/delay'],...
      |         'DelayLength', int2str(1));
      |     
      |     % Add bitslice
      |     add_block('hdlsllib/Logic and Bit Operations/Bit Slice',...
      |         [gcb, '/wr_bitslice'], 'Position',...
      |         [-65 180 25 220]);
      | 
      |     % Set bitslice parameters
      |     set_param([gcb, '/wr_bitslice'],...
      |         'lidx', int2str(ceil(log2(d)-1)));
      |     set_param([gcb, '/wr_bitslice'],...
      |         'ridx', int2str(log2(a(1))));
      |     
      |     % Add bitslice
      |     add_block('hdlsllib/Logic and Bit Operations/Bit Slice',...
      |         [gcb, '/rd_bitslice'], 'Position',...
      |         [-65 280 25 320]);
      | 
      |     % Set bitslice parameters
      |     set_param([gcb, '/rd_bitslice'],...
      |         'lidx', int2str(ceil(log2(d)-1)));
      |     set_param([gcb, '/rd_bitslice'],...
      |         'ridx', int2str(log2(a(1))));
      |     
      |     for i = 1:ceil(numbram)
      |         
      |         %%%%% Begin Adding Blocks %%%%%
      |         % Add Simple RAM
      |         add_block('hdlsllib/HDL RAMs/Simple Dual Port RAM',...
      |             [gcb, '/simple_ram_', int2str(i-1)], 'Position',...
      |             [635 0+600*y 635+200 400+600*y]);
      | 
      |         % Set RAM parameters
      |         set_param([gcb, '/simple_ram_', int2str(i-1)],...
      |             'ram_size', int2str(log2(a(1))));
      | 
      |         % Add compare to constant
      |         add_block('hdlsllib/Logic and Bit Operations/Compare To Constant',...
      |             [gcb, '/wr_cmp2const_', int2str(i-1)], 'Position',...
      |             [190 225+y*600 220 255+y*600]); 
      | 
      |         % Set compare to zero parameters
      |         set_param([gcb, '/wr_cmp2const_', int2str(i-1)],...
      |             'relop', '==');
      | 
      |         % Set compare to zero parameters
      |         set_param([gcb, '/wr_cmp2const_', int2str(i-1)],...
      |             'const', int2str(i-1));
      |         
      |         % Add compare to constant
      |         add_block('hdlsllib/Logic and Bit Operations/Compare To Constant',...
      |             [gcb, '/rd_cmp2const_', int2str(i-1)], 'Position',...
      |             [190 445+y*600 220 475+y*600]); 
      | 
      |         % Set compare to zero parameters
      |         set_param([gcb, '/rd_cmp2const_', int2str(i-1)],...
      |             'relop', '==');
      | 
      |         % Set compare to zero parameters
      |         set_param([gcb, '/rd_cmp2const_', int2str(i-1)],...
      |             'const', int2str(i-1));
      | 
      |         % Add and logic
      |         add_block('hdlsllib/Logic and Bit Operations/Logical Operator',...
      |             [gcb, '/and_', int2str(i-1)], 'Position',...
      |             [420 231+600*y 455 264+600*y]);
      | 
      |         % Set and logic parameters
      |         set_param([gcb, '/and_', int2str(i-1)],...
      |             'Operator', 'AND');
      | 
      |         % Add Switch
      |         add_block('hdlsllib/Signal Routing/Switch',...
      |             [gcb, '/switch_', int2str(i-1)], 'Position',...
      |             [685 -113+600*y 785 -37+600*y]);
      | 
      |         % Set switch parameters
      |         set_param([gcb, '/switch_', int2str(i-1)],...
      |             'Threshold', int2str(1));
      | 
      |         % Add Constant
      |         add_block('hdlsllib/Sources/Constant',...
      |             [gcb, '/constant_', int2str(i-1)], 'Position',...
      |             [425 -115+600*y 455 -85+600*y]);
      | 
      |         % Set Constant parameters
      |         set_param([gcb, '/constant_', int2str(i-1)],...
      |             'Value', int2str(i-1));
      |         set_param([gcb, '/constant_', int2str(i-1)],...
      |             'OutDataTypeStr', ['fixdt(0, ', int2str(ceil(numbram)), ', 0)']);   
      | 
      |         %%%%% Begin Wire Connections %%%%%        
      |         % Connect "wr_data" to "simple_ram_i"
      |         add_line(gcb, 'wr_data/1', ['simple_ram_', int2str(i-1), '/1'],...
      |             'autorouting','on');
      | 
      |         % Connect "wr_address" to "simple_ram_i"
      |         add_line(gcb, 'wr_address/1', ['simple_ram_', int2str(i-1), '/2'],...
      |             'autorouting','on');
      | 
      |         % Connect "rd_address" to "simple_ram_i"
      |         add_line(gcb, 'rd_address/1', ['simple_ram_', int2str(i-1), '/4'],...
      |             'autorouting','on');
      | 
      |         % Connect "constant_i" to "switch_i"
      |         add_line(gcb, ['constant_', int2str(i-1), '/1'], ['switch_', int2str(i-1), '/1'],...
      |             'autorouting','on');
      | 
      |         % Connect "zero" to "switch_i"
      |         add_line(gcb, 'zero/1', ['switch_', int2str(i-1), '/3'],...
      |             'autorouting','on');
      | 
      |         % Connect "switch_i" to "vector_concatenate"
      |         add_line(gcb, ['switch_', int2str(i-1), '/1'], ['vector_concatenate/', int2str(i)],...
      |             'autorouting','on');
      | 
      |         % Connect "rd_address" to "simple_ram_i"
      |         add_line(gcb, ['simple_ram_', int2str(i-1), '/1'], ['multiport_switch/', int2str(i+1)],...
      |             'autorouting','on');
      | 
      |         % Connect "bitslice_i" to "wr_cmp2const_i"
      |         add_line(gcb, ['wr_bitslice/1'], ['wr_cmp2const_', int2str(i-1), '/1'],...
      |             'autorouting','on');
      |         
      |         % Connect "bitslice_i" to "rd_cmp2const_i"
      |         add_line(gcb, ['rd_bitslice/1'], ['rd_cmp2const_', int2str(i-1), '/1'],...
      |             'autorouting','on');
      | 
      |         % Connect "wr_en" to "and_i"
      |         add_line(gcb, ['wr_en/1'], ['and_', int2str(i-1), '/2'],...
      |             'autorouting','on');
      | 
      |         % Connect "and_i" to "simple_ram_0"
      |         add_line(gcb, ['and_', int2str(i-1), '/1'], ['simple_ram_', int2str(i-1), '/3'],...
      |             'autorouting','on');
      | 
      |         % Connect "wr_cmp2const_i" to "and_i"
      |         add_line(gcb, ['wr_cmp2const_', int2str(i-1), '/1'], ['and_', int2str(i-1), '/1'],...
      |             'autorouting','on');
      | 
      |         % Connect "rd_cmp2const_i" to "switch_i"
      |         add_line(gcb, ['rd_cmp2const_', int2str(i-1), '/1'], ['switch_', int2str(i-1), '/2'],...
      |             'autorouting','on');
      |          
      |         % Update coordinates
      |         y = y + 1;
      |         
      |     end
      |     
      |     % Connect "rd_addr" to "bitslice_i"
      |     add_line(gcb, ['rd_addr/1'], ['rd_bitslice/1'],...
      |         'autorouting','on');
      |     
      |     % Connect "wr_addr" to "bitslice_i"
      |     add_line(gcb, ['wr_addr/1'], ['wr_bitslice/1'],...
      |         'autorouting','on');
      |     
      |     % Connect "wr_addr" to "wr_address"
      |     add_line(gcb, 'wr_addr/1', ['wr_address', '/1'],...
      |         'autorouting','on');
      | 
      |     % Connect "rd_addr" to "rd_address"
      |     add_line(gcb, 'rd_addr/1', ['rd_address', '/1'],...
      |         'autorouting','on');
      | 
      |     % Connect "vector_concatenate" to "bitwise_or"
      |     add_line(gcb, ['vector_concatenate/1'], ['bitwise_or/1'],...
      |         'autorouting','on');
      | 
      |     % Connect "bitwise_or" to "delay"
      |     add_line(gcb, ['bitwise_or/1'], ['delay/1'],...
      |         'autorouting','on');
      | 
      |     % Connect "delay" to "multiport_switch"
      |     add_line(gcb, ['delay/1'], ['multiport_switch/1'],...
      |         'autorouting','on');
      | 
      |     % Connect "multiport_switch" to "rd_data"
      |     add_line(gcb, ['multiport_switch/1'], ['rd_data/1'],...
      |         'autorouting','on');
      |     
      | end
      | 
      | % If there is a half bram we must change a few parameters. Firstly, delete
      | % the write and read address lines. Then add bitslice blocks to reduce the
      | % address space in half. Connect rd_addr and wr_addr to the corresponding ports
      | % on the bram. Finally, change the address depth.
      | if halfbram
      |     
      |     if ceil(numbram) > 1
      |         
      |         % Delete lines
      |         delete_line(gcb, ['wr_address/1'], ['simple_ram_', int2str(i-1), '/2'])
      |         delete_line(gcb, ['rd_address/1'], ['simple_ram_', int2str(i-1), '/4'])
      |         
      |         % Write Address half ram Slice
      |         add_block('hdlsllib/Logic and Bit Operations/Bit Slice',...
      |                 [gcb, '/wr_address_hr'], 'Position',...
      |                 [160 130+(y-1)*600 250 170+(y-1)*600]);
      |         % Set bitslice parameters
      |         set_param([gcb, '/wr_address_hr'],...
      |             'lidx', int2str(log2(a(1))-2));
      |         set_param([gcb, '/wr_address_hr'],...
      |             'ridx', int2str(0));
      | 
      |         % Read Address half ram Slice
      |         add_block('hdlsllib/Logic and Bit Operations/Bit Slice',...
      |                 [gcb, '/rd_address_hr'], 'Position',...
      |                 [160 330+(y-1)*600 250 370+(y-1)*600]);
      |         % Set bitslice parameters
      |         set_param([gcb, '/rd_address_hr'],...
      |             'lidx', int2str(log2(a(1))-2));
      |         set_param([gcb, '/rd_address_hr'],...
      |             'ridx', int2str(0));
      | 
      |         % Connect "wr_addr" to "wr_address_hr"
      |         add_line(gcb, 'wr_addr/1', ['wr_address_hr', '/1'],...
      |             'autorouting','on');
      | 
      |         % Connect "rd_addr" to "rd_address_hr"
      |         add_line(gcb, 'rd_addr/1', ['rd_address_hr', '/1'],...
      |             'autorouting','on');
      | 
      |         % Connect "wr_address_hr" to "simple_ram_i"
      |         add_line(gcb, ['wr_address_hr', '/1'], ['simple_ram_', int2str(i-1), '/2'],...
      |             'autorouting','on');
      | 
      |         % Connect "rd_address_hr" to "simple_ram_i"
      |         add_line(gcb, ['rd_address_hr', '/1'], ['simple_ram_', int2str(i-1), '/4'],...
      |             'autorouting','on');
      |         
      |         % Update the ram parameters (address bits)
      |         set_param([gcb, '/simple_ram_', int2str(i-1)],...
      |             'ram_size', int2str(log2(a(1)/2)));
      | 
      |     else
      |         % Set bitslice parameters
      |         % set_param([gcb, '/wr_address'],...
      |         %     'lidx', int2str(log2(a(1))-2));
      |         % set_param([gcb, '/wr_address'],...
      |         %     'ridx', int2str(0));
      |         % Set bitslice parameters
      |         % set_param([gcb, '/rd_address'],...
      |         %     'lidx', int2str(log2(a(1))-2));
      |         % set_param([gcb, '/rd_address'],...
      |         %     'ridx', int2str(0));
      |         
      |     end
      |     
      | 
      |     
      | end
  rd_data : Outport

== system lht_1280_720/DUT/LHT/Parallel LHT Kernel/Efficient Hough Kernel/Look Ahead Hough/Register Bank ==
  Input : Inport
  Enable : EnablePort
  Tapped Delay : simulink/Discrete/Tapped Delay  vinit=0  samptime=-1  NumDelays=nTheta/2  DelayOrder=Oldest  includeCurrent=on
  Output : Outport  InitialOutput=0  VectorParamsAs1DForOutWhenUnconnected=off
  wires:
  Tapped Delay/1 -> Output/1
  Input/1 -> Tapped Delay/1

== system lht_1280_720/DUT/LHT/Parallel LHT Kernel/Efficient Hough Kernel/Look Ahead Hough/Rising Edge Detector ==
  Input : Inport
  AND : Logic  IconShape=distinctive  AllPortsSameDT=off  OutDataTypeStr=boolean
  Delay : Delay  DelayLength=1
  NOT : Logic  Operator=NOT  IconShape=distinctive  AllPortsSameDT=off  OutDataTypeStr=boolean
  Output : Outport  VectorParamsAs1DForOutWhenUnconnected=off
  wires:
  AND/1 -> Output/1
  Input/1 -> AND/2, Delay/1
  Delay/1 -> NOT/1
  NOT/1 -> AND/1

== system lht_1280_720/DUT/LHT/Parallel LHT Kernel/Efficient Hough Kernel/Look Ahead Hough/sin LUT ==
  Address : Inport
  1-D Lookup Table : Lookup_n-D  NumberOfTableDimensions=1  BreakpointsForDimension1=[0:1:nTheta/2]  IndexSearchMethod=Evenly spaced points  Table=fi(sin(deg2rad(theta(1:1:nTheta/2+1))), 1, 16, 14)  InterpMethod=Flat  ExtrapMethod=Clip  DiagnosticForOutOfRangeInput=Error  InternalRulePriority=Speed  OutDataTypeStr=fixdt(1,16,14)  RndMeth=Simplest  InputSameDT=on
  sin : Outport
  wires:
  1-D Lookup Table/1 -> sin/1
  Address/1 -> 1-D Lookup Table/1

== system lht_1280_720/DUT/LHT/Parallel LHT Accumulator/Accumulator with Switches/Accumulator/Block RAM/Simple Dual Port RAM ==
  wr_data : Inport
  wr_addr : Inport  Port=2
  wr_en : Inport  Port=3
  rd_addr : Inport  Port=4
  Simple Dual Port RAM : hdlsllib/HDL RAMs/Simple Dual Port RAM  ram_size=ceil(log2(maxRho*2))
      settings: SourceProductBaseCode=SL
  rd_data : Outport
  wires:
  Simple Dual Port RAM/1 -> rd_data/1
  rd_addr/1 -> Simple Dual Port RAM/4
  wr_en/1 -> Simple Dual Port RAM/3
  wr_addr/1 -> Simple Dual Port RAM/2
  wr_data/1 -> Simple Dual Port RAM/1

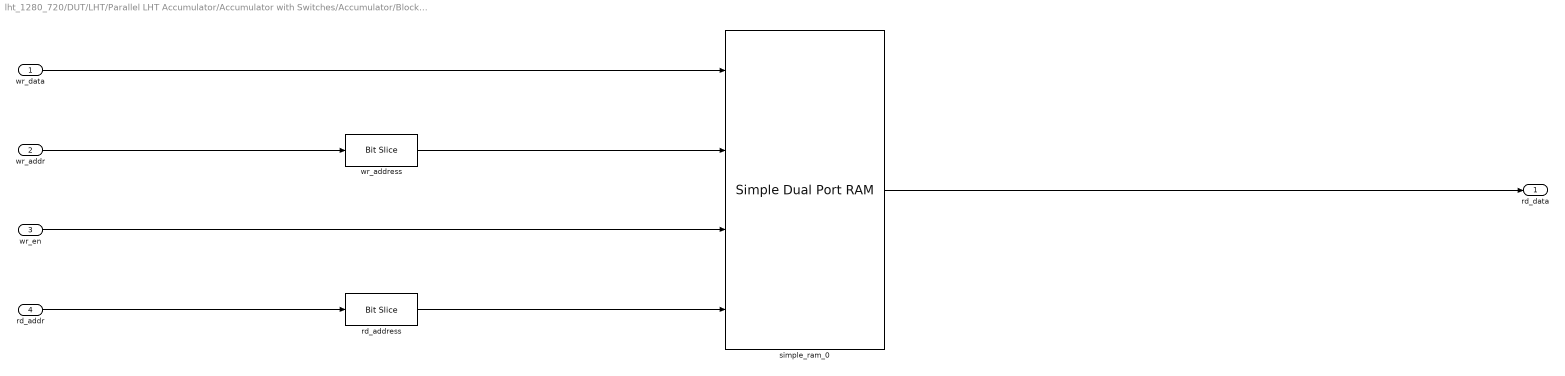
== system lht_1280_720/DUT/LHT/Parallel LHT Accumulator/Accumulator with Switches/Accumulator/Block RAM/Simple Dual Port RAM Generator ==
  wr_data : Inport
  wr_addr : Inport  Port=2
  wr_en : Inport  Port=3
  rd_addr : Inport  Port=4
  rd_address : hdlsllib/Logic and Bit Operations/Bit Slice  lidx=10  ridx=0
      settings: SourceProductBaseCode=SL
  simple_ram_0 : hdlsllib/HDL RAMs/Simple Dual Port RAM  ram_size=11
      settings: SourceProductBaseCode=SL
  wr_address : hdlsllib/Logic and Bit Operations/Bit Slice  lidx=10  ridx=0
      settings: SourceProductBaseCode=SL
  rd_data : Outport
  wires:
  wr_data/1 -> simple_ram_0/1
  wr_addr/1 -> wr_address/1
  wr_address/1 -> simple_ram_0/2
  wr_en/1 -> simple_ram_0/3
  rd_addr/1 -> rd_address/1
  rd_address/1 -> simple_ram_0/4
  simple_ram_0/1 -> rd_data/1
